simulink model "signal_generation_mdl"  (R2022b)
settings: Solver=FixedStepDiscrete  StartTime=0.0  StopTime=inf  FixedStep=0.0001  RelTol=1e-3
undefined symbols (not defined in the file): allSignals, signalIDs
settings Model: Creator=adelk  LastModifiedBy=adelk

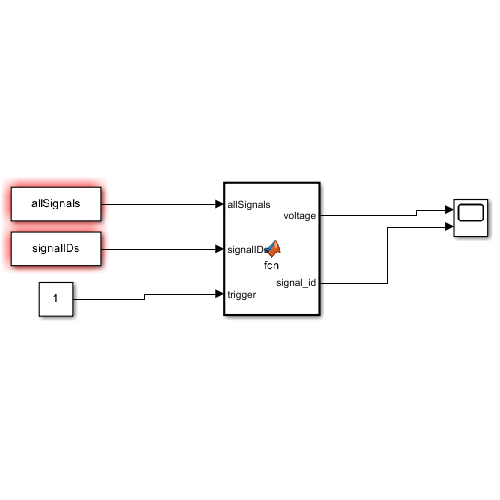
[thumbnail: Simulink's stored preview of the top-level diagram]
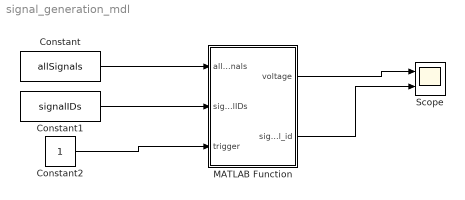
== system signal_generation_mdl ==
  Constant : Constant  Value=allSignals
  Constant1 : Constant  Value=signalIDs
  Constant2 : Constant
  MATLAB Function : MATLAB Function  TreatAsAtomicUnit=on
  Scope : Scope  NumInputPorts=2
  wires:
  Constant/1 -> MATLAB Function/1(allSignals)
  MATLAB Function/1(voltage) -> Scope/1
  Constant1/1 -> MATLAB Function/2(signalIDs)
  Constant2/1 -> MATLAB Function/3(trigger)
  MATLAB Function/2(signal_id) -> Scope/2

== matlab function signal_generation_mdl/MATLAB Function ==
  data: allSignals input; signalIDs input; voltage output; trigger input; signal_id output
function [voltage, signal_id] = fcn(allSignals, signalIDs, trigger)

persistent idx

if (isempty(idx))
    idx = 0;
end

if trigger 
    idx = idx + 1;

    if idx > length(allSignals)
        idx = length(allSignals);
    end
    
    voltage = allSignals(idx);
    signal_id = signalIDs(idx);
else
    voltage = 0;
    signal_id = 0;
end
